simulink model "teta_2wbr"  (R2017b)
settings: Solver=VariableStepAuto  StartTime=0.0  StopTime=10.0  RelTol=1e-3
libraries: simulink_extras x3, simulink x1
settings Model: Creator=Iman  LastModifiedBy=Iman

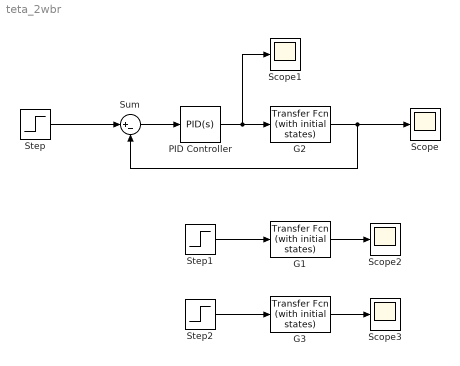
== system teta_2wbr ==
  G1 : simulink_extras/Additional Linear/Transfer Fcn (with initial states)  N="[-1.932e04   4.666e07  2.734e12  5.557e15  4.591e17  2.648e06].*(-1)"  D="[1  5372   2.732e08  1.366e12  1.934e16  8.664e19  1.019e23  -7.863e21 5.559e24 0 ]"  X0=0
  G2 : simulink_extras/Additional Linear/Transfer Fcn (with initial states)  N="[-1.932e04 -1.666e06  -2.309e-06].*(-1)"  D="[1 3043  1.324e08  3.695e11  -1.875e10  -2.01e13]"  X0=0
  G3 : simulink_extras/Additional Linear/Transfer Fcn (with initial states)  N="[-1.932e04 -1.666e06  -2.309e-06].*(-1)"  D="[1 3043  1.324e08  3.695e11  -1.875e10  -2.01e13]"  X0=0
  PID Controller : simulink/Continuous/PID Controller  Controller=PID  TimeDomain=Continuous-time  SampleTime=-1  IntegratorMethod=Forward Euler  FilterMethod=Forward Euler  Form=Parallel  UseFilter=on  ControllerParametersSource=internal  P=-19090877.2850556  I=-49314002.2069424  D=-1374600.36376171  N=28.947665758353  InitialConditionSource=internal  InitialConditionForIntegrator=0  InitialConditionForFilter=0  ExternalReset=none  LimitOutput=off  UpperSaturationLimit=inf  LowerSaturationLimit=-inf  LinearizeAsGain=on  AntiWindupMode=none  Kb=1  TrackingMode=off  Kt=1  PParamMin=[]  PParamMax=[]  IParamMin=[]  IParamMax=[]  DParamMin=[]  DParamMax=[]  NParamMin=[]  NParamMax=[]  KbParamMin=[]  KbParamMax=[]  KtParamMin=[]  KtParamMax=[]  POutMin=[]  POutMax=[]  IOutMin=[]  IOutMax=[]  DOutMin=[]  DOutMax=[]  NOutMin=[]  NOutMax=[]  KbOutMin=[]  KbOutMax=[]  KtOutMin=[]  KtOutMax=[]  IntegratorOutMin=[]  IntegratorOutMax=[]  FilterOutMin=[]  FilterOutMax=[]  SumOutMin=[]  SumOutMax=[]  SumI1OutMin=[]  SumI1OutMax=[]  SumI2OutMin=[]  SumI2OutMax=[]  SumI3OutMin=[]  SumI3OutMax=[]  SumDOutMin=[]  SumDOutMax=[]  SaturationOutMin=[]  SaturationOutMax=[]  IntegratorContinuousStateAttributes=''  IntegratorStateMustResolveToSignalObject=off  IntegratorRTWStateStorageClass=Auto  FilterContinuousStateAttributes=''  FilterStateMustResolveToSignalObject=off  FilterRTWStateStorageClass=Auto  DifferentiatorICPrevScaledInput=0  DifferentiatorOutMin=[]  DifferentiatorOutMax=[]  InitialConditionSetting=State (most efficient)  FilterDiffOutCoefMin=[]  FilterDiffOutCoefMax=[]  SumDenOutMin=[]  SumDenOutMax=[]  SumNumOutMin=[]  SumNumOutMax=[]  ReciprocalOutMin=[]  ReciprocalOutMax=[]  DivideOutMin=[]  DivideOutMax=[]  TunerSelectOption=Transfer Function Based (PID Tuner App)
  Scope{,1..3} (4 alike) : Scope
  Step : Step  Time=0  SampleTime=0
  Step1 : Step  Time=0  SampleTime=0
  Step2 : Step  Time=0  SampleTime=0
  Sum : Sum  Inputs=|+-
  wires:
  PID Controller/1 -> G2/1, Scope1/1
  G2/1 -> Sum/2, Scope/1
  Sum/1 -> PID Controller/1
  Step/1 -> Sum/1
  G1/1 -> Scope2/1
  Step1/1 -> G1/1
  Step2/1 -> G3/1
  G3/1 -> Scope3/1
